simulink model "open_loop_complet_system"  (R2022a)
settings: Solver=ode45  StartTime=0.0  StopTime=10.0  RelTol=1e-3  EnableMultiTasking=on
values from neighbouring files (symbols this model uses):
  Jpl = 0.0124    [lead_compensator.m]    (also in open_loop_complete_system_analysis.m; poles_placement_kp_kv.m; poles_placement_kp_kv_int.m)
  Jw = Jpl/100    (= 0.000124)    [lead_compensator.m]    (also in open_loop_complete_system_analysis.m; poles_placement_kp_kv.m; poles_placement_kp_kv_int.m)
  ke = 0.0001    [lead_compensator.m]    (also in open_loop_complete_system_analysis.m; poles_placement_kp_kv.m; poles_placement_kp_kv_int.m)
  ki = 1    [lead_compensator.m]    (also in open_loop_complete_system_analysis.m; poles_placement_kp_kv.m; poles_placement_kp_kv_int.m)
  km = 0.0235    [lead_compensator.m]    (also in open_loop_complete_system_analysis.m; poles_placement_kp_kv.m; poles_placement_kp_kv_int.m)
  L = 0.050    (= 0.05)    [lead_compensator.m]    (also in open_loop_complete_system_analysis.m; poles_placement_kp_kv.m; poles_placement_kp_kv_int.m)
  R = 9.7    [lead_compensator.m]    (also in open_loop_complete_system_analysis.m; poles_placement_kp_kv.m; poles_placement_kp_kv_int.m)
settings Model: Creator=c.berard  LastModifiedBy=fades
settings SolverCC: AlgebraicLoopSolver=TrustRegion
settings DataIOCC: LimitDataPoints=on  SaveFormat=Array  SignalLoggingSaveFormat=ModelDataLogs  ReturnWorkspaceOutputs=off  SignalLoggingName=sigsOut
settings OptimizationCC: ExpressionDepthLimit=2147483647  LifeSpan=inf
settings DebuggingCC: SaveWithParameterizedLinksMsg=none  UnderspecifiedInitializationDetection=Classic  MergeDetectMultiDrivingBlocksExec=none  SignalResolutionControl=TryResolveAllWithWarning  MultiTaskDSMMsg=warning  MultiTaskCondExecSysMsg=none  FcnCallInpInsideContextMsg=warning  UnconnectedInputMsg=warning  UnconnectedOutputMsg=warning  UnconnectedLineMsg=warning  StateNameClashWarn=warning  SFUnexpectedBacktrackingDiag=warning  SFNoUnconditionalDefaultTransitionDiag=warning  SFExecutionAtInitializationDiag=none  SFMachineParentedDataDiag=warning  ArithmeticOperatorsInVariantConditions=warning
settings HardwareCC: ProdBitPerPointer=32  ProdBitPerSizeT=32  ProdBitPerPtrDiffT=32  ProdLargestAtomicFloat=None  ProdIntDivRoundTo=Undefined  ProdEndianess=Unspecified  ProdWordSize=32  ProdHWDeviceType=32-bit Generic  TargetUnknown=on
settings ModelReferenceCC: PropagateSignalLabelsOutOfModel=off
settings SFSimCC: SimUseLocalCustomCode=off  CustomCodeUndefinedFunction=UseInterfaceOnly
settings RTWCC: RTWUseLocalCustomCode=off
settings CodeAppCC: StateflowObjectComments=on
settings GRTTargetCC: TargetLangStandard=C89/C90 (ANSI)  CombineOutputUpdateFcns=off  GRTInterface=on
settings ConfigComp: CovMetricSettings=dw  CovSaveCumulativeToWorkspaceVar=on  CovSaveSingleToWorkspaceVar=on  CovExternalEMLEnable=off

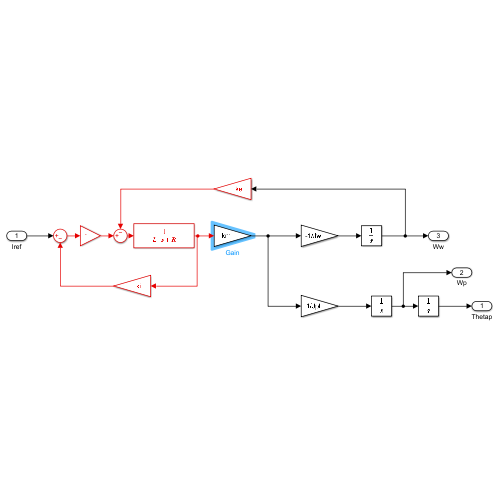
[thumbnail: Simulink's stored preview of the top-level diagram]
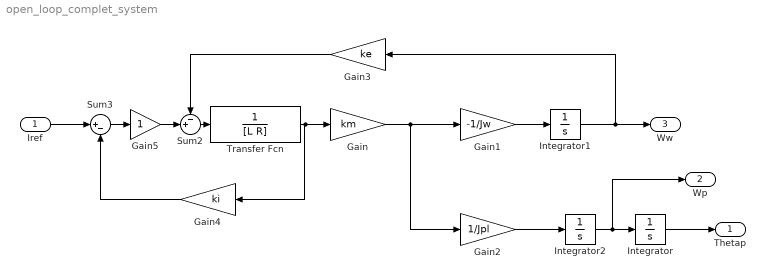
== system open_loop_complet_system ==
  "Iref " : Inport
  Gain : Gain  Gain=km  SaturateOnIntegerOverflow=on  OutDataTypeStr=Inherit: Same as input  ParamDataTypeStr=Inherit: Same as input
  Gain1 : Gain  Gain=-1/Jw  SaturateOnIntegerOverflow=on  OutDataTypeStr=Inherit: Same as input  ParamDataTypeStr=Inherit: Same as input
  Gain2 : Gain  Gain=1/Jpl  SaturateOnIntegerOverflow=on  OutDataTypeStr=Inherit: Same as input  ParamDataTypeStr=Inherit: Same as input
  Gain3 : Gain  Gain=ke  SaturateOnIntegerOverflow=on  OutDataTypeStr=Inherit: Same as input  ParamDataTypeStr=Inherit: Same as input
  Gain4 : Gain  Gain=ki  SaturateOnIntegerOverflow=on  OutDataTypeStr=Inherit: Same as input  ParamDataTypeStr=Inherit: Same as input
  Gain5 : Gain
  Integrator : Integrator
  Integrator1 : Integrator
  Integrator2 : Integrator
  Sum2 : Sum  Inputs=-+|
  Sum3 : Sum  Inputs=|+-
  Transfer Fcn : TransferFcn  Denominator=[L R]
  Thetap : Outport
  Wp : Outport  Port=2
  Ww : Outport  Port=3
  wires:
  Gain1/1 -> Integrator1/1
  Gain2/1 -> Integrator2/1
  Integrator2/1 -> Wp/1, Integrator/1
  Integrator1/1 -> Ww/1, Gain3/1
  Integrator/1 -> Thetap/1
  Gain/1 -> Gain2/1, Gain1/1
  Transfer Fcn/1 -> Gain/1, Gain4/1
  Sum2/1 -> Transfer Fcn/1
  Sum3/1 -> Gain5/1
  Gain3/1 -> Sum2/1
  Gain4/1 -> Sum3/2
  "Iref "/1 -> Sum3/1
  Gain5/1 -> Sum2/2
